simulink model "FunzioneDinamicaInversaSimulink"  (R2020b)
settings: Solver=VariableStepAuto  StartTime=0.0  StopTime=1  RelTol=1e-3
values from neighbouring files (symbols this model uses):
  theta1ldm = theta1 + Ldm_theta1.moto.data{1,1}.v    [PKM_main.m]
  theta1ldm_p = theta1_p + Ldm_theta1.moto.data{2,1}.v    [PKM_main.m]
  theta2ldm = theta2 + Ldm_theta2.moto.data{1,1}.v    [PKM_main.m]
  theta2ldm_p = theta2_p + Ldm_theta2.moto.data{2,1}.v    [PKM_main.m]
settings Model: Creator=daniele_ravasio  LastModifiedBy=daniele_ravasio

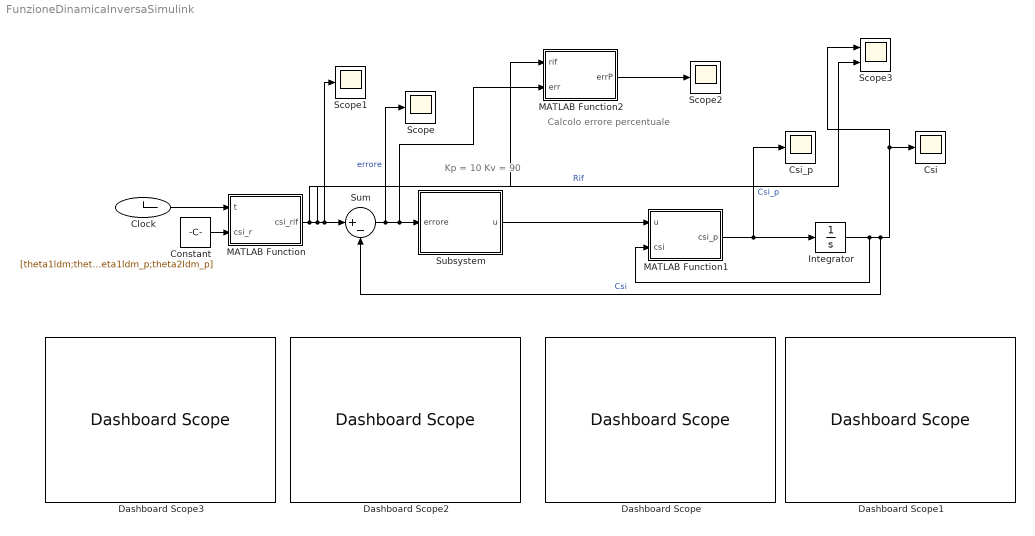
== system FunzioneDinamicaInversaSimulink ==
  note: Calcolo errore percentuale
  note: Kp = 10
      | Kv = 90
  Clock : Clock
  Constant : Constant  Value=[theta1ldm;theta2ldm;theta1ldm_p;theta2ldm_p]  VectorParams1D=off
  Csi : Scope
  Csi_p : Scope
  Dashboard Scope : DashboardScope
  Dashboard Scope1 : DashboardScope
  Dashboard Scope2 : DashboardScope  Ymin=-2  Ymax=2
  Dashboard Scope3 : DashboardScope
  Integrator : Integrator  InitialCondition=[theta1ldm(1,1);theta2ldm(1,1);theta1ldm_p(1,1);theta2ldm_p(1,1)]
  MATLAB Function : MATLAB Function  TreatAsAtomicUnit=on
  MATLAB Function1 : MATLAB Function  TreatAsAtomicUnit=on
  MATLAB Function2 : MATLAB Function  TreatAsAtomicUnit=on
  Scope : Scope
  Scope1 : Scope
  Scope2 : Scope
  Scope3 : Scope  NumInputPorts=2
  Subsystem : Subsystem
  Sum : Sum  Inputs=|+-
  wires:
  Integrator/1 -> Sum/2, Scope3/1, Csi/1, MATLAB Function1/2(csi)  "Csi"
  MATLAB Function1/1(csi_p) -> Integrator/1, Csi_p/1  "Csi_p"
  Sum/1 -> MATLAB Function2/2(err), Subsystem/1(errore), Scope/1  "errore"
  Clock/1 -> MATLAB Function/1(t)
  Subsystem/1(u) -> MATLAB Function1/1(u)
  Constant/1 -> MATLAB Function/2(csi_r)
  MATLAB Function/1(csi_rif) -> MATLAB Function2/1(rif), Scope3/2, Scope1/1, Sum/1  "Rif"
  MATLAB Function2/1(errP) -> Scope2/1

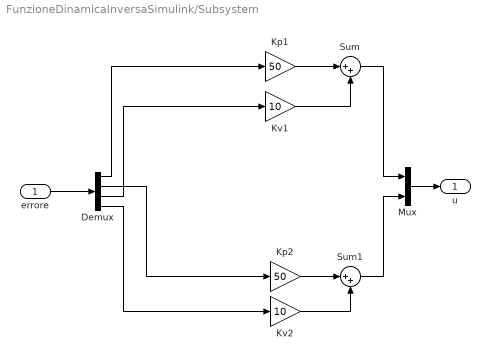
== system FunzioneDinamicaInversaSimulink/Subsystem ==
  errore : Inport
  Demux : Demux
  Kp1 : Gain  Gain=50
  Kp2 : Gain  Gain=50
  Kv1 : Gain  Gain=10
  Kv2 : Gain  Gain=10
  Mux : Mux  Inputs=2
  Sum : Sum  Inputs=|++
  Sum1 : Sum  Inputs=|++
  u : Outport
  wires:
  errore/1 -> Demux/1
  Demux/1 -> Kp1/1
  Demux/4 -> Kv2/1
  Mux/1 -> u/1
  Demux/3 -> Kv1/1
  Demux/2 -> Kp2/1
  Kp1/1 -> Sum/1
  Kv1/1 -> Sum/2
  Sum/1 -> Mux/1
  Kp2/1 -> Sum1/1
  Kv2/1 -> Sum1/2
  Sum1/1 -> Mux/2

== matlab function FunzioneDinamicaInversaSimulink/MATLAB Function ==
  data: t input; csi_rif output; csi_r input
function csi_rif = fcn(t,csi_r)


% tempo T, f(T), tempo di interpolazione (t) 
T = linspace(0,1,1000);
csi_rif = [interp1(T,csi_r(1,:),t);interp1(T,csi_r(2,:),t);interp1(T,csi_r(3,:),t);interp1(T,csi_r(4,:),t)];
%y_cap(2,:) = interp1(T,Tau(2,:),t);

== matlab function FunzioneDinamicaInversaSimulink/MATLAB Function2 ==
  data: rif input; errP output; err input
function errP = fcn(rif,err)

errP = (err./rif)*100;

== matlab function FunzioneDinamicaInversaSimulink/MATLAB Function1 ==
  data: u input; csi_p output; csi input
function csi_p = f(u,csi)

csi_p = F(u,csi);
